simulink model "EurlerDynJointVerifyIdn"  (Simulink 7.6)
settings: Solver=ode45  StartTime=0.0  StopTime=8  RelTol=1e-3
InitFcn:
  | eval('Config')
values from neighbouring files (symbols this model uses):
  a2 = 0    [Config.m]    (also in CtrPlatformCfg.m)
  a3 = 0    [Config.m]    (also in CtrPlatformCfg.m)
  a4 = 0    [Config.m]    (also in CtrPlatformCfg.m)
  a5 = 90    [Config.m]    (also in CtrPlatformCfg.m)
  a6 = 0    [Config.m]    (also in CtrPlatformCfg.m)
  DH_EU = [266     300     0       0       1016     0      174 ... (first row only)    [DynEulerTest.m]
  freq = tvel/radius    (= 1)    [Config.m]    (also in CtrPlatformCfg.m)
  Ft_EU = [0;0;0;0;0;0]    [DynEulerTest.m]
  init_Endx = gd_init(1,4)    [Config.m]    (also in CtrPlatformCfg.m)
  init_Endy = gd_init(2,4)    [Config.m]    (also in CtrPlatformCfg.m)
  init_Endz = gd_init(3,4)    [Config.m]    (also in CtrPlatformCfg.m)
  init_Rot = gd_init(1:3,1:3)    [Config.m]    (also in CtrPlatformCfg.m)
  L = [l1 l2 l3 l4 l5 l6 l7 l8 l9]    [Config.m]    (also in CtrPlatformCfg.m)
  tvel = 120    [Config.m]    (also in CtrPlatformCfg.m)
undefined symbols (not defined in the file or in its folder): a1, DH_Min, Ft_Min, Param_EU, Param_Min
libraries: mblibv1 x35, simulink x9
(part 2 of 2)

== system EurlerDynJointVerifyIdn/Circle_YZ/EndVelocity ==
  Constant : Constant  Value=-1
  End_Vx : Constant  Value=0
  End_Vy : Sin  Frequency=freq  Phase=pi/2  SampleTime=0
  End_Vz : Sin  Amplitude=-tvel  Frequency=freq  SampleTime=0
  Gain : Gain  Gain=tvel
  Ramp : simulink/Sources/Ramp  SystemSampleTime=-1  slope=1  start=0  X0=0
  Ramp1 : simulink/Sources/Ramp  SystemSampleTime=-1  slope=-1  start=1  X0=0
  Sum : Sum  Inputs=|++
  Sum1 : Sum  Inputs=++|
  Sum2 : Sum  Inputs=++|
  Transport Delay : TransportDelay
  Transport Delay1 : TransportDelay
  EndVx : Outport
  EndVy : Outport  Port=2
  EndVz : Outport  Port=3
  wires:
  End_Vy/1 -> Sum2/1
  Ramp/1 -> Sum/1
  Ramp1/1 -> Sum/2
  Transport Delay/1 -> Sum1/1
  Sum2/1 -> Transport Delay/1
  Constant/1 -> Sum2/2
  Sum/1 -> Sum1/2
  Sum1/1 -> Gain/1
  End_Vz/1 -> Transport Delay1/1
  Gain/1 -> EndVy/1
  Transport Delay1/1 -> EndVz/1
  End_Vx/1 -> EndVx/1

== system EurlerDynJointVerifyIdn/Line/EndVelocity ==
  End_Vx : Constant  Value=30
  End_Vy : Constant  Value=30
  End_Vz : Constant  Value=-30
  EndVx : Outport
  EndVy : Outport  Port=2
  EndVz : Outport  Port=3
  wires:
  End_Vx/1 -> EndVx/1
  End_Vz/1 -> EndVz/1
  End_Vy/1 -> EndVy/1

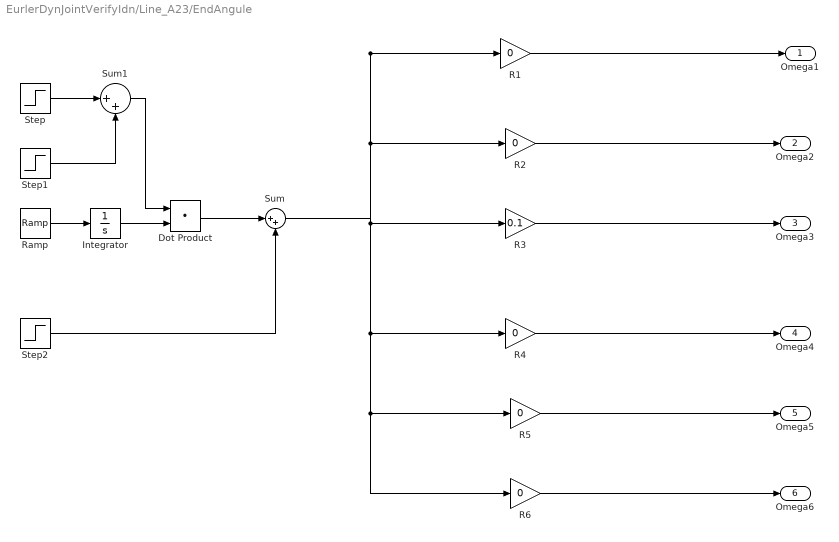
== system EurlerDynJointVerifyIdn/Line_A23/EndAngule ==
  Dot Product : DotProduct  InputSameDT=on  OutDataTypeStr=Inherit: Inherit via internal rule
  Integrator : Integrator
  R{1..2,4..6} (5 alike) : Gain  Gain=0
  R3 : Gain  Gain=0.1
  Ramp : simulink/Sources/Ramp  SystemSampleTime=-1  slope=1  start=0  X0=0
  Step : Step  After=-2  SampleTime=0
  Step1 : Step  Time=0  After=2  SampleTime=0
  Step2 : Step  SampleTime=0
  Sum : Sum  Inputs=|++
  Sum1 : Sum  Inputs=|++
  Omega1 : Outport
  Omega2 : Outport  Port=2
  Omega3 : Outport  Port=3
  Omega4 : Outport  Port=4
  Omega5 : Outport  Port=5
  Omega6 : Outport  Port=6
  wires:
  Step1/1 -> Sum1/2
  Step2/1 -> Sum/2
  Dot Product/1 -> Sum/1
  Sum1/1 -> Dot Product/1
  Step/1 -> Sum1/1
  Integrator/1 -> Dot Product/2
  Sum/1 -> R6/1, R5/1, R4/1, R3/1, R2/1, R1/1
  R1/1 -> Omega1/1
  Ramp/1 -> Integrator/1
  R2/1 -> Omega2/1
  R3/1 -> Omega3/1
  R5/1 -> Omega5/1
  R6/1 -> Omega6/1
  R4/1 -> Omega4/1

== system EurlerDynJointVerifyIdn/Line_Acc/EndAcc ==
  End_Vx : Constant  Value=0
  End_Vy : Constant  Value=0
  End_Vz : Constant  Value=0
  EndAccx : Outport
  EndAccy : Outport  Port=2
  EndAccz : Outport  Port=3
  wires:
  End_Vy/1 -> EndAccy/1
  End_Vz/1 -> EndAccz/1
  End_Vx/1 -> EndAccx/1

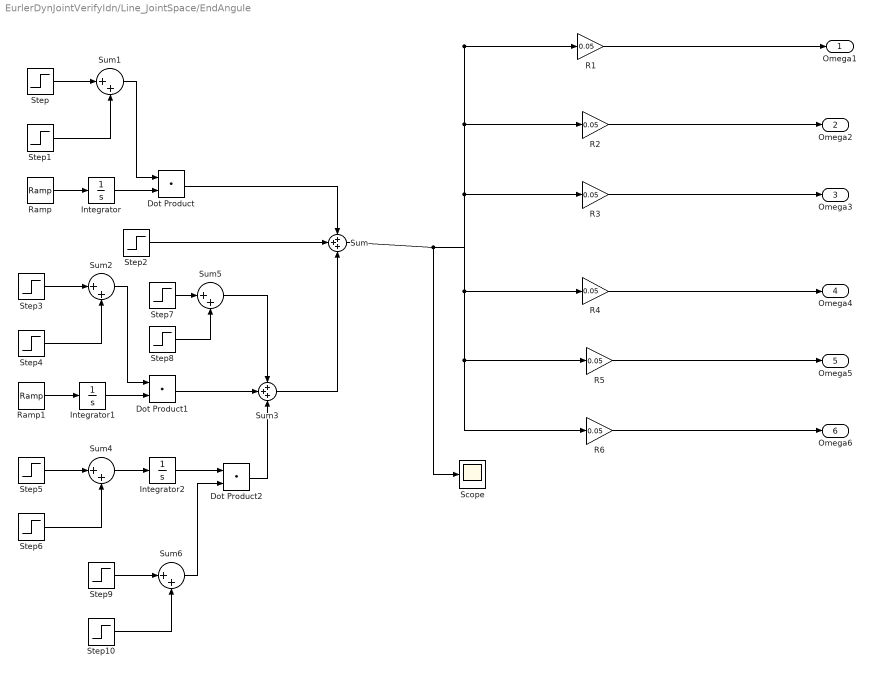
== system EurlerDynJointVerifyIdn/Line_JointSpace/EndAngule ==
  Dot Product : DotProduct  InputSameDT=on  OutDataTypeStr=Inherit: Inherit via internal rule
  Dot Product1 : DotProduct  InputSameDT=on  OutDataTypeStr=Inherit: Inherit via internal rule
  Dot Product2 : DotProduct  InputSameDT=on  OutDataTypeStr=Inherit: Inherit via internal rule
  Integrator : Integrator
  Integrator1 : Integrator
  Integrator2 : Integrator
  R{1..6} (6 alike) : Gain  Gain=0.05
  Ramp : simulink/Sources/Ramp  SystemSampleTime=-1  slope=1  start=0  X0=0
  Ramp1 : simulink/Sources/Ramp  SystemSampleTime=-1  slope=-1  start=0  X0=0
  Scope : Scope
      settings: SaveName=ScopeData21
  Step : Step  After=-1  SampleTime=0
  Step1 : Step  Time=0  SampleTime=0
  Step10 : Step  SampleTime=0
  Step2 : Step  Time=2  SampleTime=0
  Step3 : Step  Time=2  After=-1  SampleTime=0
  Step4 : Step  SampleTime=0
  Step5 : Step  Time=2  After=-2  SampleTime=0
  Step6 : Step  After=2  SampleTime=0
  Step7 : Step  Time=2  After=-1  SampleTime=0
  Step8 : Step  SampleTime=0
  Step9 : Step  Time=2  After=-1  SampleTime=0
  Sum : Sum  Inputs=+++
  Sum{1..2,4..6} (5 alike) : Sum  Inputs=|++
  Sum3 : Sum  Inputs=+++
  Omega1 : Outport
  Omega2 : Outport  Port=2
  Omega3 : Outport  Port=3
  Omega4 : Outport  Port=4
  Omega5 : Outport  Port=5
  Omega6 : Outport  Port=6
  wires:
  R4/1 -> Omega4/1
  R6/1 -> Omega6/1
  R5/1 -> Omega5/1
  R3/1 -> Omega3/1
  R2/1 -> Omega2/1
  Ramp/1 -> Integrator/1
  R1/1 -> Omega1/1
  Sum/1 -> R1/1, R2/1, R3/1, R4/1, R5/1, R6/1, Scope/1
  Integrator/1 -> Dot Product/2
  Step/1 -> Sum1/1
  Sum1/1 -> Dot Product/1
  Step1/1 -> Sum1/2
  Dot Product/1 -> Sum/1
  Step2/1 -> Sum/2
  Ramp1/1 -> Integrator1/1
  Integrator1/1 -> Dot Product1/2
  Step3/1 -> Sum2/1
  Sum2/1 -> Dot Product1/1
  Step4/1 -> Sum2/2
  Sum3/1 -> Sum/3
  Step5/1 -> Sum4/1
  Step6/1 -> Sum4/2
  Sum4/1 -> Integrator2/1
  Dot Product1/1 -> Sum3/2
  Step7/1 -> Sum5/1
  Step8/1 -> Sum5/2
  Sum5/1 -> Sum3/1
  Step9/1 -> Sum6/1
  Step10/1 -> Sum6/2
  Integrator2/1 -> Dot Product2/1
  Sum6/1 -> Dot Product2/2
  Dot Product2/1 -> Sum3/3

== system EurlerDynJointVerifyIdn/Still/EndVelocity ==
  Constant : Constant  Value=0
  Constant1 : Constant  Value=0
  Constant2 : Constant  Value=0
  EndVx : Outport
  EndVy : Outport  Port=2
  EndVz : Outport  Port=3
  wires:
  Constant/1 -> EndVx/1
  Constant1/1 -> EndVy/1
  Constant2/1 -> EndVz/1

== matlab function Circle_XY/Jacobian ==
  data: Omega output double; EndVel input double; Theta input double; L parameter double
function Omega = fcn(EndVel,Theta,L)
%#eml

Omega = zeros(6,1);
V = [EndVel; 0; 0; 0];   
g = fwd_kin(L,Theta');
Jb = body_Jacobian(L,Theta');
Adg_inv = double(AdjointInv(g));
Omega = double((Jb \ Adg_inv* V)')';

== matlab function Circle_XY/Inverse Kinematic ==
  data: EndPos input double; init_Rot parameter double; theta output double; L parameter double
function theta = fcn(EndPos,init_Rot,L)
%#eml
theta =[0;0; 0; 0; 0; 0];
gd = [init_Rot,EndPos;[0 0 0],1];
[theta_total,num_total] = inv_kin(gd,L);
theta = theta_total(:,2);

== matlab function Dynamic Euler/Newton Euler Recursion ==
  data: Pos input double; Torque output double; Vel input double; Acc input double; DH_EU parameter double; Param_EU parameter double; Ft_EU parameter double
function Torque = fcn(Pos,Vel,Acc,DH_EU,Param_EU,Ft_EU)
%#eml
Torque = [0;0;0;0;0;0];
Torque = DynEulerCal(DH_EU,Param_EU,Ft_EU,Pos,Vel,Acc);

== matlab function Circle_XZ/Inverse Kinematic ==
  data: EndPos input double; init_Rot parameter double; theta output double; L parameter double
function theta = fcn(EndPos,init_Rot,L)
%#eml
theta =[0;0; 0; 0; 0; 0];
gd = [init_Rot,EndPos;[0 0 0],1];
[theta_total,num_total] = inv_kin(gd,L);
theta = theta_total(:,2);

== matlab function Circle_XZ/Jacobian ==
  data: Omega output double; EndVel input double; Theta input double; L parameter double
function Omega = fcn(EndVel,Theta,L)
%#eml

Omega = zeros(6,1);
V = [EndVel; 0; 0; 0];   
g = fwd_kin(L,Theta');
Jb = body_Jacobian(L,Theta');
Adg_inv = double(AdjointInv(g));
Omega = double((Jb \ Adg_inv* V)')';

== matlab function Line_A23/Forward ==
  data: Theta input double; EndPos output double; L parameter double
function EndPos = fcn(Theta,L)
%#eml
gd = fwd_kin(L,Theta');
EndPos = gd(1:3,4);

== matlab function Line_A23/Jacobian ==
  data: Theta input double; Omega input double; EndVel output double; L parameter double
function EndVel = fcn(Theta,Omega,L)
%#eml


EndVW = spat_Jacobian(L,Theta')*Omega;
gd = fwd_kin(L,Theta');
EndW = EndVW(4:6,1);
gd_pos = gd(1:3,4);
EndVel=cross(EndW,gd_pos);

== matlab function Line_Acc/Inverse Kinematic ==
  data: EndPos input double; init_Rot parameter double; theta output double; L parameter double
function theta = fcn(EndPos,init_Rot,L)
%#eml
theta =[0;0; 0; 0; 0; 0];
gd = [init_Rot,EndPos;[0 0 0],1];
[theta_total,num_total] = inv_kin(gd,L);
theta = theta_total(:,2);

== matlab function Line_Acc/Jacobian ==
  data: Omega output double; EndVel input double; Theta input double; L parameter double
function Omega = fcn(EndVel,Theta,L)
%#eml

Omega = zeros(6,1);
V = [EndVel; 0; 0; 0];   
g = fwd_kin(L,Theta');
Jb = body_Jacobian(L,Theta');
Adg_inv = double(AdjointInv(g));
Omega = double((Jb \ Adg_inv* V)')';

== matlab function Circle_YZ/Inverse Kinematic ==
  data: EndPos input double; init_Rot parameter double; theta output double; L parameter double
function theta = fcn(EndPos,init_Rot,L)
%#eml
theta =[0;0; 0; 0; 0; 0];
gd = [init_Rot,EndPos;[0 0 0],1];
[theta_total,num_total] = inv_kin(gd,L);
theta = theta_total(:,2);

== matlab function Circle_YZ/Jacobian ==
  data: Omega output double; EndVel input double; Theta input double; L parameter double
function Omega = fcn(EndVel,Theta,L)
%#eml

Omega = zeros(6,1);
V = [EndVel; 0; 0; 0];   
g = fwd_kin(L,Theta');
Jb = body_Jacobian(L,Theta');
Adg_inv = double(AdjointInv(g));
Omega = double((Jb \ Adg_inv* V)')';

== matlab function Line_JointSpace/Forward ==
  data: Theta input double; EndPos output double; L parameter double
function EndPos = fcn(Theta,L)
%#eml
gd = fwd_kin(L,Theta');
EndPos = gd(1:3,4);

== matlab function Line_JointSpace/Jacobian ==
  data: Theta input double; Omega input double; EndVel output double; L parameter double
function EndVel = fcn(Theta,Omega,L)
%#eml


EndVW = spat_Jacobian(L,Theta')*Omega;
gd = fwd_kin(L,Theta');
EndW = EndVW(4:6,1);
gd_pos = gd(1:3,4);
EndVel=cross(EndW,gd_pos);

== matlab function Still/Inverse Kinematic ==
  data: EndPos input double; init_Rot parameter double; theta output double; L parameter double
function theta = fcn(EndPos,init_Rot,L)
%#eml
theta =[0;0; 0; 0; 0; 0];
gd = [init_Rot,EndPos;[0 0 0],1];
[theta_total,num_total] = inv_kin(gd,L);
theta = theta_total(:,2);

== matlab function Still/Jacobian ==
  data: Omega output double; EndVel input double; Theta input double; L parameter double
function Omega = fcn(EndVel,Theta,L)
%#eml

Omega = zeros(6,1);
V = [EndVel; 0; 0; 0];   
g = fwd_kin(L,Theta');
Jb = body_Jacobian(L,Theta');
Adg_inv = double(AdjointInv(g));
Omega = double((Jb \ Adg_inv* V)')';

== matlab function Line/Inverse Kinematic ==
  data: EndPos input double; init_Rot parameter double; theta output double; L parameter double
function theta = fcn(EndPos,init_Rot,L)
%#eml
theta =[0;0; 0; 0; 0; 0];
gd = [init_Rot,EndPos;[0 0 0],1];
[theta_total,num_total] = inv_kin(gd,L);
theta = theta_total(:,2);

== matlab function Line/Jacobian ==
  data: Omega output double; EndVel input double; Theta input double; L parameter double
function Omega = fcn(EndVel,Theta,L)
%#eml

Omega = zeros(6,1);
V = [EndVel; 0; 0; 0];   
g = fwd_kin(L,Theta');
Jb = body_Jacobian(L,Theta');
Adg_inv = double(AdjointInv(g));
Omega = double((Jb \ Adg_inv* V)')';

== matlab function Joint/Forward ==
  data: Theta input double; EndPos output double; L parameter double
function EndPos = fcn(Theta,L)
%#eml
gd = fwd_kin(L,Theta');
EndPos = gd(1:3,4);

== matlab function Joint/Jacobian ==
  data: Theta input double; Omega input double; EndVel output double; L parameter double
function EndVel = fcn(Theta,Omega,L)
%#eml


EndVW = spat_Jacobian(L,Theta')*Omega;
gd = fwd_kin(L,Theta');
EndW = EndVW(4:6,1);
gd_pos = gd(1:3,4);
EndVel=cross(EndW,gd_pos);

== matlab function Dynamic Euler/Newton Euler Recursion1 ==
  data: Pos input double; Torque output double; Vel input double; Acc input double; DH_Min parameter double; Param_Min parameter double; Ft_Min parameter double
function Torque = fcn(Pos,Vel,Acc,DH_Min,Param_Min, Ft_Min)
%#eml
Torque = [0;0;0;0;0;0];
Torque = DynEulerCal_Min(DH_Min,Param_Min,Ft_Min,Pos,Vel,Acc);
